simulink model "Drone2_simulink_old"  (R2024b)
settings: Solver=ode1be  StartTime=0.0  StopTime=1200  FixedStep=0.001  MaxStep=0.001  MinStep=0.00095  RelTol=1e-3
undefined symbols (not defined in the file): DiscIntNeverNeededParam, Environment, Newton, Raphson, Sim3dSensor, Vehicle, X, Y, Z
libraries: sm_lib x2953, nesl_utility x76, slpidlib x25, simulink x4, eeGeneralControl x4, matrix_library x3, rllib x2, sim3dlib x2, uavsim3dlib x2, dspstat3 x1, SignalEditorBlockLib x1, sharedutil x1
(part 1 of 21)
settings Model: Creator=Robotics  LastModifiedBy=admin
settings SolverCC: InitialStep=0.00095  MaxConsecutiveMinStep=5  ZeroCrossAlgorithm=Adaptive  EnableFixedStepZeroCrossing=on
settings OptimizationCC: ZeroExternalMemoryAtStartup=off  ZeroInternalMemoryAtStartup=off  InitFltsAndDblsToZero=on
settings DebuggingCC: AlgebraicLoopMsg=none
settings HardwareCC: ProdLongLongMode=on  TargetLongLongMode=on
settings RTWCC: TargetLang=C++  GenerateGPUCode=CUDA
settings GRTTargetCC: TargetLangStandard=C++11 (ISO)  CodeInterfacePackaging=C++ class
settings ExplorerConfigSet: InternalSimMechanicsExplorerSettings="<ExplorerConfiguration><canonicalview>default</canonicalview><AnimationSetting><BasePlaybackSpeed>1.0</BasePlaybackSpeed><PlaybackSpeedFactor>4.0</PlaybackSpeedFactor></AnimationSetting><TilePanel><TileInfo><Tiles Columns=\"2\" Count=\"4\" Rows=\"2\"><Column Weight=\"0.5\"/><Column Weight=\"0.5\"/><Row Weight=\"0.499\"/><Row Weight=\"0.501\"/><Tile Height=\"1\" Width=\"1\" X=\"0\" Y=\"0\"/><Tile Height=\"1\" Width=\"1\" X=\"0\" Y=\"1\"/><Tile Height=\"1\" Width=\"1\" X=\"1\" Y=\"0\"/><Tile Height=\"1\" Width=\"1\" X=\"1\" Y=\"1\"/></Tiles></TileInfo><SceneInfo><SceneViewer><BGColor><R>0.60000002384185791</R><G>0.60000002384185791</G><B>0.60000002384185791</B></BGColor><Camera><DoPerspective>off</DoPerspective><Position><X>-0.0113675484149264941</X><Y>-739.397084901340122</Y><Z>-0.0886193408787913639</Z></Position><Center><X>-0.0113675484149264941</X><Y>-5.95973369854618626e-06</Y><Z>-0.0886193408787913639</Z></Center><Up><X>0</X><Y>-0</Y><Z>1</Z></Up><ViewLimDist>1</ViewLimDist><YLim>0.330538852611916067</YLim><XLim>0.39239407649250857</XLim></Camera></SceneViewer><SceneViewer><BGColor><R>0.60000002384185791</R><G>0.60000002384185791</G><B>0.60000002384185791</B></BGColor><Camera><DoPerspective>off</DoPerspective><Position><X>-0.0123326458289036989</X><Y>0.0124784466883283152</Y><Z>779.159585012589673</Z></Position><Center><X>-0.0123326458289036989</X><Y>0.0124784466883283152</Y><Z>-5.16521799909241963e-06</Z></Center><Up><X>0</X><Y>1</Y><Z>-0</Z></Up><ViewLimDist>1</ViewLimDist><YLim>0.581385630746349302</YLim><XLim>0.686170250241330937</XLim></Camera></SceneViewer><SceneViewer><BGColor><R>0.60000002384185791</R><G>0.60000002384185791</G><B>0.60000002384185791</B></BGColor><Camera><DoPerspective>off</DoPerspective><Position><X>779.159585093457963</X><Y>0.0121540939985229218</Y><Z>-0.0872146397947211049</Z></Position><Center><X>-1.32520503939304035e-05</X><Y>0.0121540939985229218</Y><Z>-0.0872146397947211049</Z></Center><Up><X>-0</X><Y>0</Y><Z>1</Z></Up><ViewLimDist>1</ViewLimDist><YLim>0.279113201164486624</YLim><XLim>0.331344911323922742</XLim></Camera></SceneViewer><SceneViewer><BGColor><R>0.60000002384185791</R><G>0.60000002384185791</G><B>0.60000002384185791</B></BGColor><Camera><DoPerspective>off</DoPerspective><Position><X>436.235740070213467</X><Y>-436.218598621418209</Y><Z>436.235051594773893</Z></Position><Center><X>-13.3273814067072021</X><Y>13.344522855502376</Y><Z>-13.3280698821460408</Z></Center><Up><X>-0.408248290463863073</X><Y>0.408248290463863073</Y><Z>0.816496580927726145</Z></Up><ViewLimDist>1</ViewLimDist><YLim>0.509054047074245841</YLim><XLim>0.600802160209720437</XLim></Camera></SceneViewer></SceneInfo></TilePanel><MechEditorPanel><Cameras><Camera><Id>Camera1</Id><Value><Name>Camera1</Name><NativeCamera><PositionTrackingFeature>Physical_system.camera.F</PositionTrackingFeature><CenterTrackingFeature>Physical_system.camera.F</CenterTrackingFeature><UpVectorTrackingFeature>Physical_system.camera.F</UpVectorTrackingFeature><CenterTrackingOrigin>off</CenterTrackingOrigin><CenterTrackingDirection>+X</CenterTrackingDirection><UpVectorTrackingDirection>+Z</UpVectorTrackingDirection></NativeCamera></Value></Camera></Cameras><GfxPanelCameraMap/><VideoCreator><PlaybackSpeedRatio>8.0</PlaybackSpeedRatio><FrameRate>60</FrameRate><VideoFormat>Motion JPEG AVI</VideoFormat><FrameSize>[1920 1080]</FrameSize></VideoCreator></MechEditorPanel></ExplorerConfiguration>"

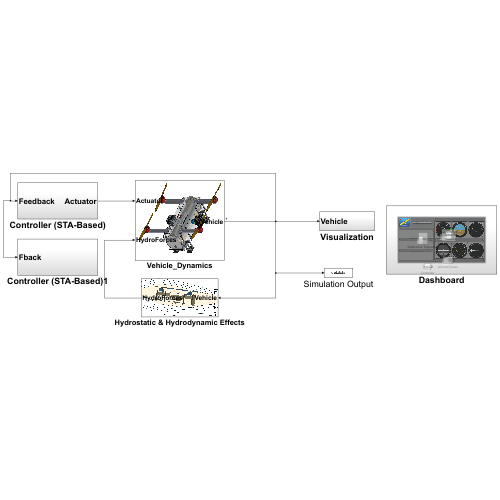
[thumbnail: Simulink's stored preview of the top-level diagram]
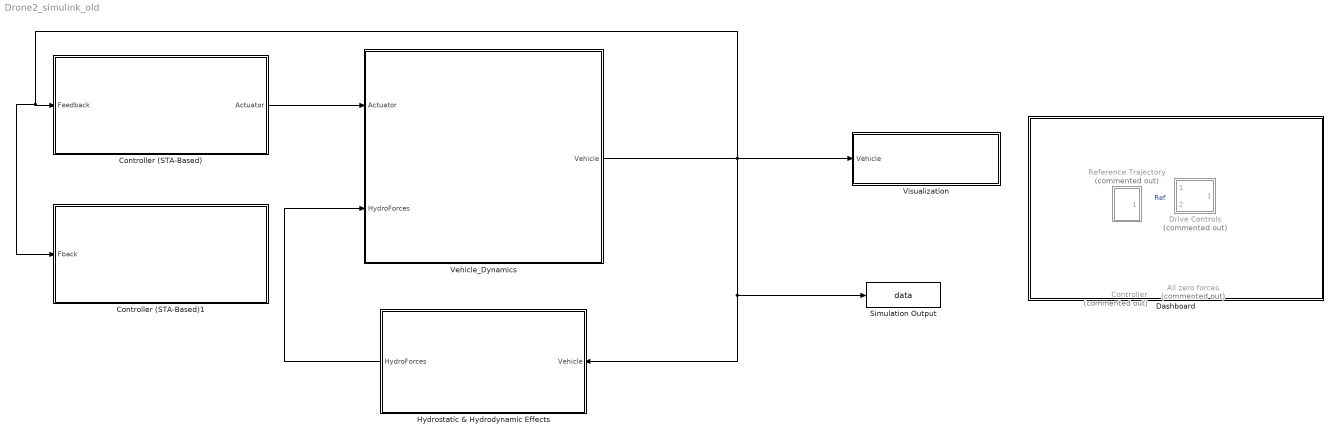
== system Drone2_simulink_old ==
  All zero forces : Subsystem  Commented=on
  Controller : Subsystem  Commented=on
  Controller (STA-Based) : Subsystem
  Controller (STA-Based)1 : Subsystem
  Dashboard : Subsystem
  Drive Controls : Subsystem  Commented=on
  Hydrostatic & Hydrodynamic Effects : Subsystem
      mask Display: image('Drage_new.png', [0,0,0,0,95,95])
  Reference Trajectory : Subsystem  Commented=on
  Simulation Output : ToWorkspace  VariableName=data  SaveFormat=Timeseries  SampleTime=-1
  Vehicle_Dynamics : Subsystem
      mask Display: image('Drone2_Assembly.PNG');
  Visualization : Subsystem
  wires:
  Reference Trajectory/1(Reference) -> Drive Controls/2(Reference)  "Ref"
  Vehicle_Dynamics/1(Vehicle) -> Hydrostatic & Hydrodynamic Effects/1(Vehicle), Simulation Output/1, Controller (STA-Based)1/1(Fback), Controller (STA-Based)/1(Feedback), Visualization/1(Vehicle)
  Hydrostatic & Hydrodynamic Effects/1(HydroForces) -> Vehicle_Dynamics/2(HydroForces)
  Controller (STA-Based)/1(Actuator) -> Vehicle_Dynamics/1(Actuator)

== system Drone2_simulink_old/All zero forces ==
  Constant : Constant  Value=0
  Constant3 : Constant  Value=0
  Constant9 : Constant  Value=0
  Out Bus Element : Outport  PortName=Actuator  Element=Aerial.MotorRB.Thrust
  Out Bus Element1 : Outport  PortName=Actuator  Element=Aerial.MotorRB.Torque
  Out Bus Element2 : Outport  PortName=Actuator  Element=Aerial.MotorRF.Torque
  Out Bus Element5 : Outport  PortName=Actuator  Element=Aerial.MotorRF.Thrust
  Out Bus Element3 : Outport  PortName=Actuator  Element=Aerial.MotorLF.Torque
  Out Bus Element6 : Outport  PortName=Actuator  Element=Aerial.MotorLF.Thrust
  Out Bus Element4 : Outport  PortName=Actuator  Element=Aerial.MotorLB.Torque
  Out Bus Element7 : Outport  PortName=Actuator  Element=Aerial.MotorLB.Thrust
  Out Bus Element8 : Outport  PortName=Actuator  Element=Underwater.ThrusterL.Thrust
  Out Bus Element9 : Outport  PortName=Actuator  Element=Underwater.ThrusterL.Torque
  Out Bus Element10 : Outport  PortName=Actuator  Element=Underwater.ThrusterR.Torque
  Out Bus Element11 : Outport  PortName=Actuator  Element=Underwater.ThrusterR.Thrust
  Out Bus Element12 : Outport  PortName=Actuator  Element=BuoyancyForce.SyringeFL.Force
  Out Bus Element13 : Outport  PortName=Actuator  Element=BuoyancyForce.SyringeFR.Force
  Out Bus Element14 : Outport  PortName=Actuator  Element=BuoyancyForce.SyringeB.Force
  wires:
  Constant/1 -> Out Bus Element9/1, Out Bus Element10/1
  Constant3/1 -> Out Bus Element11/1, Out Bus Element8/1
  Constant9/1 -> Out Bus Element13/1, Out Bus Element12/1, Out Bus Element14/1, Out Bus Element5/1, Out Bus Element2/1, Out Bus Element/1, Out Bus Element1/1, Out Bus Element6/1, Out Bus Element3/1, Out Bus Element7/1, Out Bus Element4/1

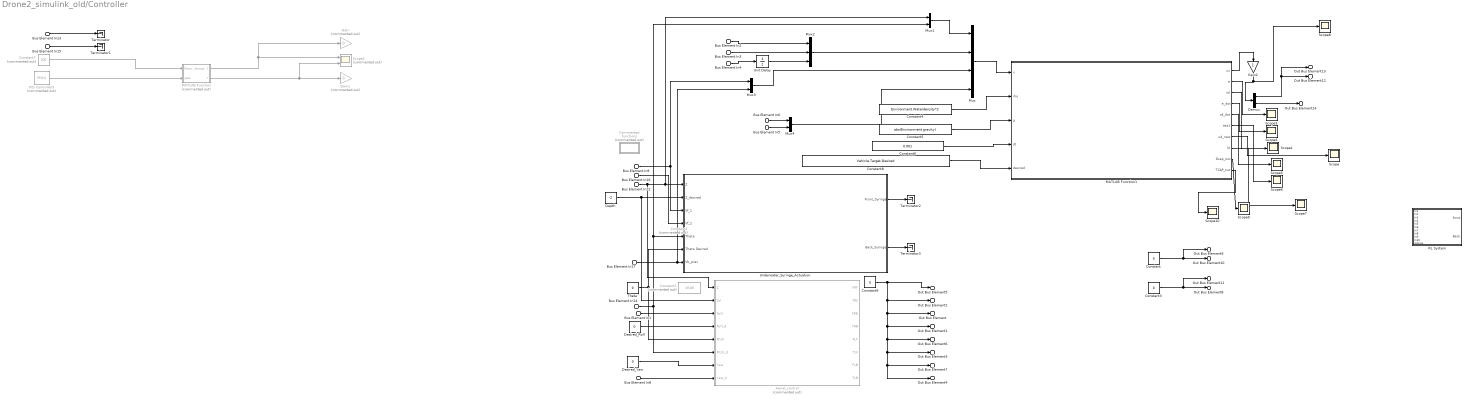
== system Drone2_simulink_old/Controller ==
  Bus Element In17 : Inport  PortName=Feedback  Element=Buoyancy.Syringe.SyringeB.Pose
  Bus Element In5 : Inport  PortName=Feedback  Element=Buoyancy.Syringe.SyringeB.Vel
  Bus Element In9 : Inport  PortName=Feedback  Element=Buoyancy.Syringe.SyringeFR.Pose
  Bus Element In6 : Inport  PortName=Feedback  Element=Buoyancy.Syringe.SyringeFR.Vel
  Bus Element In16 : Inport  PortName=Feedback  Element=Buoyancy.Syringe.SyringeFL.Pose
  Bus Element In14 : Inport  PortName=Feedback  Element=COM.Derived.Euler.theta
  Bus Element In8 : Inport  PortName=Feedback  Element=COM.Derived.Euler.psi
  Bus Element In1 : Inport  PortName=Feedback  Element=COM.Derived.Euler.phi
  Bus Element In13 : Inport  PortName=Feedback  Element=COM.World.Ve.Vz
  Bus Element In12 : Inport  PortName=Feedback  Element=COM.World.Xe.Z
  Bus Element In15 : Inport  PortName=Feedback  Element=COM.Body.wb.q
  Bus Element In2 : Inport  PortName=Feedback  Element=COM.Body.Vb.u
  Bus Element In3 : Inport  PortName=Feedback  Element=COM.Body.Vb.w
  Bus Element In4 : Inport  PortName=Feedback  Element=COM.Body.dwbdt.qdot
  Aerial_control : Subsystem  Commented=on
  Commented functions : Subsystem  Commented=on
  Constant : Constant  Value=0
  Constant1 : Constant  Commented=on  Value=19.85
  Constant2 : Constant  Commented=on  Value=20
  Constant3 : Constant  Value=0
  Constant4 : Constant  Value=Environment.Waterdensity*2
  Constant5 : Constant  Value=abs(Environment.gravity)
  Constant6 : Constant  Value=0.001
  Constant7 : Constant  Commented=on  Value=100
  Constant8 : Constant  Value=Vehicle.Target.Desired
  Constant9 : Constant  Value=0
  Demux : Demux  Outputs=2
  Depth : Constant  Value=-2
  Desired_Roll : Constant  Value=0
  Desired_Yaw : Constant  Value=0
  Gain : Gain  Commented=on  Gain=0
  Gain1 : Gain  Commented=on  Gain=0
  Gain2 : Gain
  MATLAB Function : MATLAB Function  Commented=on  TreatAsAtomicUnit=on
  MATLAB Function1 : MATLAB Function  TreatAsAtomicUnit=on
  Mux : Mux
  Mux1 : Mux  Inputs=2
  Mux2 : Mux  Inputs=3
  Mux3 : Mux  Inputs=2
  Mux4 : Mux  Inputs=2
  PID Controller3 : slpidlib/PID Controller  Commented=on  Controller=PD  Form=Parallel  TimeDomain=Discrete-time  UseExternalTs=off  SampleTime=0.001  IntegratorMethod=Forward Euler  FilterMethod=Backward Euler  ControllerParametersSource=internal  P=100  I=1  UseKiTs=off  D=5  UseExternalDerivativeSource=off  N=100  UseFilter=on  TunerSelectOption=Transfer Function Based (PID Tuner App)  InitialConditionSource=internal  InitialConditionForIntegrator=0  InitialConditionForFilter=0  DifferentiatorICPrevScaledInput=0  ExternalReset=none  TrackingMode=off  Kt=1  LimitOutput=off  SatLimitsSource=internal  UpperSaturationLimit=inf  LowerSaturationLimit=-inf  LinearizeAsGain=on  AntiWindupMode=none  Kb=1  LimitIntegrator=off  UpperIntegratorSaturationLimit=inf  LowerIntegratorSaturationLimit=-inf  POutMin=[]  POutMax=[]  IOutMin=[]  IOutMax=[]  DOutMin=[]  DOutMax=[]  NOutMin=[]  NOutMax=[]  SumOutMin=[]  SumOutMax=[]  SaturationOutMin=[]  SaturationOutMax=[]  PParamMin=[]  PParamMax=[]  IParamMin=[]  IParamMax=[]  DParamMin=[]  DParamMax=[]  NParamMin=[]  NParamMax=[]  KbParamMin=[]  KbParamMax=[]  KtParamMin=[]  KtParamMax=[]  KbOutMin=[]  KbOutMax=[]  KtOutMin=[]  KtOutMax=[]  IntegratorOutMin=[]  IntegratorOutMax=[]  FilterOutMin=[]  FilterOutMax=[]  SumI1OutMin=[]  SumI1OutMax=[]  SumI2OutMin=[]  SumI2OutMax=[]  SumI3OutMin=[]  SumI3OutMax=[]  SumI4OutMin=[]  SumI4OutMax=[]  SumDOutMin=[]  SumDOutMax=[]  DifferentiatorOutMin=[]  DifferentiatorOutMax=[]  FilterDiffOutCoefMin=[]  FilterDiffOutCoefMax=[]  ReciprocalOutMin=[]  ReciprocalOutMax=[]  SumDenOutMin=[]  SumDenOutMax=[]  SumNumOutMin=[]  SumNumOutMax=[]  DivideOutMin=[]  DivideOutMax=[]  UdiffTsProdOutMin=[]  UdiffTsProdOutMax=[]  NTsProdOutMin=[]  NTsProdOutMax=[]  UintegralTsProdOutMin=[]  UintegralTsProdOutMax=[]  UngainTsProdOutMin=[]  UngainTsProdOutMax=[]  ClampingZeroOutDataTypeStr=Inherit: Inherit via back propagation  ClampingZeroOutMin=[]  ClampingZeroOutMax=[]  FilterDenConstantOutDataTypeStr=Inherit: Inherit via back propagation  FilterDenConstantOutMin=[]  FilterDenConstantOutMax=[]  PCopyOutDataTypeStr=Inherit: Inherit via back propagation  PCopyOutMin=[]  PCopyOutMax=[]  NCopyOutDataTypeStr=Inherit: Inherit via back propagation  NCopyOutMin=[]  NCopyOutMax=[]  IntegratorContinuousStateAttributes=''  IntegratorStateMustResolveToSignalObject=off  IntegratorRTWStateStorageClass=Auto  FilterContinuousStateAttributes=''  FilterStateMustResolveToSignalObject=off  FilterRTWStateStorageClass=Auto  ParallelPVariant=InternalParameters  IdealPVariant=Disabled  IVariant=Disabled  DVariant=InternalParameters  IntegratorVariant=Disabled  SatVariant=Disabled  AWVariant=Disabled  PCopyVariant=Disabled  TRVariant=Disabled  FdbkBlocksVariant=Forward  IdealPFdbkVariant=Disabled  SatFdbkVariant=Disabled  DerivativeFilterVariant=BackwardEulerFilter  NVariant=InternalParameters  NCopyVariant=InternalParameters  FilterICVariant=InternalICsFilter  IntegratorICVariant=Disabled  ExternalResetVariant=Disabled  TRSumVariant=Passthrough  SumFdbkVariant=Disabled  SumVariant=Sum_PD  TsampFilterVariant=InternalTs  TsampNgainVariant=Passthrough  TsampIntegralVariant=Disabled_SignalSpec  ExternalSaturationOutDataTypeStr=Inherit: Same as second input  DerivativeSourceVariant=ErrorSignal
  RL System : Subsystem
  Scope{,1,3..10} (10 alike) : Scope
  Scope2 : Scope  Commented=on  NumInputPorts=2
  Terminator{,1..3} (4 alike) : Terminator
  Theta : Constant  Value=0
  Underwater_Syringe_Actuation : Subsystem
  Unit Delay : UnitDelay  SampleTime=-1  HasFrameUpgradeWarning=on
  Out Bus Element : Outport  PortName=Actuator  Element=Aerial.MotorRB.Thrust
  Out Bus Element1 : Outport  PortName=Actuator  Element=Aerial.MotorRB.Torque
  Out Bus Element2 : Outport  PortName=Actuator  Element=Aerial.MotorRF.Torque
  Out Bus Element5 : Outport  PortName=Actuator  Element=Aerial.MotorRF.Thrust
  Out Bus Element3 : Outport  PortName=Actuator  Element=Aerial.MotorLF.Torque
  Out Bus Element6 : Outport  PortName=Actuator  Element=Aerial.MotorLF.Thrust
  Out Bus Element4 : Outport  PortName=Actuator  Element=Aerial.MotorLB.Torque
  Out Bus Element7 : Outport  PortName=Actuator  Element=Aerial.MotorLB.Thrust
  Out Bus Element8 : Outport  PortName=Actuator  Element=Underwater.ThrusterL.Thrust
  Out Bus Element9 : Outport  PortName=Actuator  Element=Underwater.ThrusterL.Torque
  Out Bus Element10 : Outport  PortName=Actuator  Element=Underwater.ThrusterR.Torque
  Out Bus Element11 : Outport  PortName=Actuator  Element=Underwater.ThrusterR.Thrust
  Out Bus Element12 : Outport  PortName=Actuator  Element=BuoyancyForce.SyringeFL.Force
  Out Bus Element13 : Outport  PortName=Actuator  Element=BuoyancyForce.SyringeFR.Force
  Out Bus Element14 : Outport  PortName=Actuator  Element=BuoyancyForce.SyringeB.Force
  wires:
  Constant3/1 -> Out Bus Element8/1, Out Bus Element11/1
  Bus Element In15/1 -> Terminator1/1
  Bus Element In17/1 -> Mux3/2, Underwater_Syringe_Actuation/7(Vb_prev)
  Constant7/1 -> MATLAB Function/1(Forwardthrust)
  Constant/1 -> Out Bus Element10/1, Out Bus Element9/1
  PID Controller3/1 -> MATLAB Function/2(yaw)
  MATLAB Function/2(r) -> Gain1/1, Scope2/2
  Bus Element In16/1 -> Underwater_Syringe_Actuation/4(Vf_2)
  Bus Element In9/1 -> Mux3/1, Underwater_Syringe_Actuation/3(Vf_1)
  Bus Element In13/1 -> Terminator/1
  Bus Element In12/1 -> Mux1/1, Underwater_Syringe_Actuation/1(Z), Aerial_control/1(Z)
  Depth/1 -> Aerial_control/2(Zd), Underwater_Syringe_Actuation/2(Z_desired)
  Theta/1 -> Underwater_Syringe_Actuation/6(Theta Desired), Aerial_control/5(Pitch)
  Bus Element In14/1 -> Underwater_Syringe_Actuation/5(Theta), Mux1/2, Aerial_control/6(Pitch_d)
  Bus Element In1/1 -> Aerial_control/3(Roll)
  Desired_Roll/1 -> Aerial_control/4(Roll_d)
  Desired_Yaw/1 -> Aerial_control/7(Yaw)
  Bus Element In8/1 -> Aerial_control/8(Yaw_d)
  MATLAB Function/1(l) -> Scope2/1, Gain/1
  Constant9/1 -> Out Bus Element4/1, Out Bus Element7/1, Out Bus Element3/1, Out Bus Element6/1, Out Bus Element1/1, Out Bus Element/1, Out Bus Element2/1, Out Bus Element5/1
  Mux1/1 -> Mux/1
  Bus Element In2/1 -> Mux2/1
  Bus Element In3/1 -> Mux2/2
  Bus Element In4/1 -> Unit Delay/1
  Mux2/1 -> Mux/2
  Bus Element In5/1 -> Mux4/2
  Bus Element In6/1 -> Mux4/1
  Constant4/1 -> MATLAB Function1/2(rho)
  Constant5/1 -> MATLAB Function1/3(g)
  Constant6/1 -> MATLAB Function1/4(dt)
  Constant8/1 -> MATLAB Function1/5(desired)
  MATLAB Function1/1(uc) -> Gain2/1
  Mux/1 -> MATLAB Function1/1(x)
  Mux3/1 -> Mux/3
  Mux4/1 -> Mux/4
  Unit Delay/1 -> Mux2/3
  Underwater_Syringe_Actuation/2(Back_Syringe) -> Terminator3/1
  Underwater_Syringe_Actuation/1(Front_Syringe) -> Terminator2/1
  MATLAB Function1/3(vd) -> Scope1/1
  MATLAB Function1/2(e) -> Scope3/1
  MATLAB Function1/4(e_dot) -> Scope4/1
  MATLAB Function1/5(vd_dot) -> Scope5/1
  MATLAB Function1/6(eta1) -> Scope6/1
  Gain2/1 -> Scope8/1, Demux/1
  Demux/1 -> Out Bus Element13/1, Out Bus Element12/1
  Demux/2 -> Out Bus Element14/1
  MATLAB Function1/8(ld) -> Scope7/1
  MATLAB Function1/7(ud_new) -> Scope/1
  MATLAB Function1/9(Dcap_out) -> Scope9/1
  MATLAB Function1/10(TCAP_out) -> Scope10/1

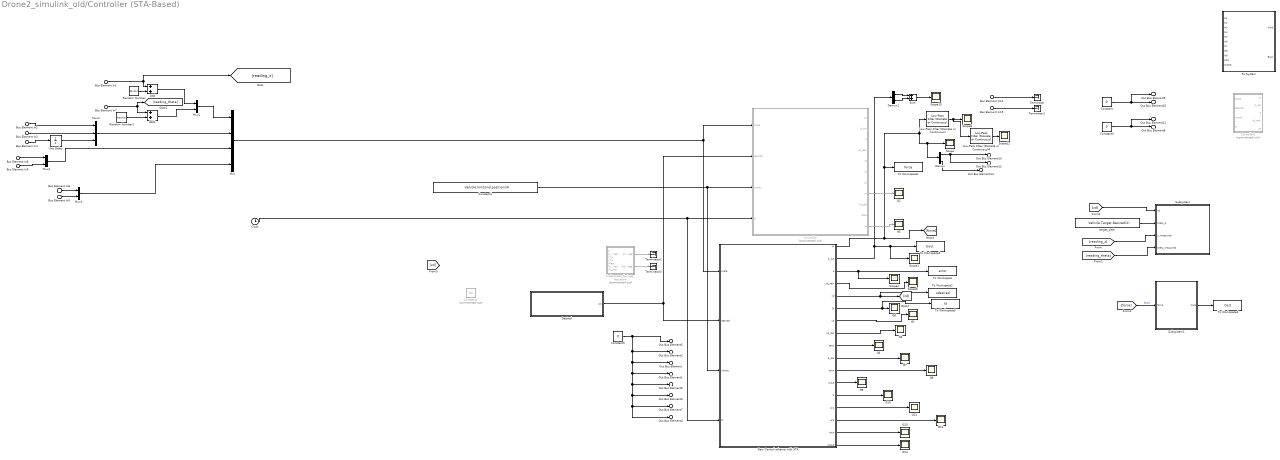
== system Drone2_simulink_old/Controller (STA-Based) ==
  Bus Element In5 : Inport  PortName=Feedback  Element=Buoyancy.Syringe.SyringeB.Vel
  Bus Element In9 : Inport  PortName=Feedback  Element=Buoyancy.Syringe.SyringeB.Pose
  Bus Element In6 : Inport  PortName=Feedback  Element=Buoyancy.Syringe.SyringeFR.Vel
  Bus Element In8 : Inport  PortName=Feedback  Element=Buoyancy.Syringe.SyringeFR.Pose
  Bus Element In13 : Inport  PortName=Feedback  Element=COM.World.Ve.Vz
  Bus Element In3 : Inport  PortName=Feedback  Element=COM.World.Ve.Vz
  Bus Element In1 : Inport  PortName=Feedback  Element=COM.World.Xe.Z
  Bus Element In15 : Inport  PortName=Feedback  Element=COM.Body.wb.q
  Bus Element In2 : Inport  PortName=Feedback  Element=COM.Body.Vb.u
  Bus Element In4 : Inport  PortName=Feedback  Element=COM.Body.dwbdt.qdot
  Bus Element In7 : Inport  PortName=Feedback  Element=COM.Derived.Euler.theta
  Add : Sum
  Add1 : Sum
  Clock : Clock
  Constant : Constant  Value=0
  Constant1 : Constant  Value=Vehicle.InitCond.position(3)
  Constant2 : Constant  Commented=on  Value=20
  Constant3 : Constant  Value=0
  Constant9 : Constant  Value=0
  Controller : MATLAB Function  Commented=on  TreatAsAtomicUnit=on  mask{m=7.61, IB=diag([0.09331 0.1703 0.2266]), Rsyringe=0.02, l=0.45, RG=[-0.002;0;-0.005], rb=[0;0;0.008], rho=Environment.Waterdensity, g=Environment.gravity, MaxBuoyancyVol=Vehicle.MaxBuoyancyForce/(abs(Environment.gravity*Environment.Waterdensity)), ZS=[0.033;0.033;0.033], Sden=1, dt=0.001, Ctrlchoice=Backsteppeng with disturbance compensator, k1e1=5, k1e2=2.5, k2e1=1, k2e2=10, k2e3=1, lambda11=5, lambda21=1, lambda12=2.5, lambda22=1, alpha1=3, KS11=01, KS12=100, KS13=10, k3e1=600, k3e2=600, TT=Vehicle.Syringe.Damping/Vehicle.Syringe.Stiffness, g1=5, g2=5, g3=5, d1=5, d2=5, sigma=0.5, sigma1=0.05, lb=0.1*eye(2), KS21=0.25, KS31=0.5, KS22=0.75, KS32=1, KS23=0.25, KS33=0.5, MaxIter=10, lambdaLM0=1e-3, tol_r=1e-6, tol_beta=1e-6, maxb=0.1, minb=0.01, alpha=0.960}
      mask prompts: m "Mass (Kg)"; IB "Inertia Matrix"; Rsyringe "Syringe radius (m)"; l "Length of Vehicle"; RG "Distance of CG from CO"; rb "Distance of CB from CO"; rho "Density"; g "Gravity"; MaxBuoyancyVol "Volume"; ZS "Syringe Z details"; Sden "Syringe Density multiplier"; dt "Sample time"; Ctrlchoice "Controller type"; k1e1 "K11"; k1e2 "K12"; k2e1 "K21"; k2e2 "K22"; k2e3 "K23"; lambda11 "lambda1-11"; lambda21 "lambda2-11"; lambda12 "lambda1-22"; lambda22 "lambda2-22"; alpha1 "STA alpha"; KS11 "KS1-11"; KS12 "KS1-22"; KS13 "KS1-33"; k3e1 "K31"; k3e2 "K32"; TT "Time constasnt"; g1 "Gamma1"; g2 "Gamma2"; g3 "Gamma3"; d1 "Delta1"; d2 "delta2"; sigma1 "T adptive sigma"; lb "Lambda b"; KS21 "KS2-11"; KS31 "KS3-11"; KS22 "KS2-22"; KS32 "KS3-22"; KS23 "KS2-33"; KS33 "KS3-33"; MaxIter "Max iteration"; lambdaLM0 "Lambda LM0"; tol_r "Relative Tolerance"; tol_beta "Beta tolerance"; maxb "Max"; minb "Min"; alpha "Smoothing constant"
      mask init:
      | % k1e1= 1; k1e2 = 1;
      | parameter.Backcomp.K1e = diag([k1e1 k1e2]); %2x2
      | 
      | % k2e1 = 10; k2e2 = 100; k2e3 =100;
      | parameter.Backcomp.K2eta1 = diag([k2e2 k2e3]); %2x2
      | 
      | % k3e1 = 200; k3e2 = 200;
      | parameter.Backcomp.K3eta2 = diag([k3e1 k3e2]);
      | 
      | % d1 = 5; d2 =5;
      | parameter.Backcomp.Del = diag([d1 d2]); %2x2
      | 
      | % g1 = 5; g2 = 5; g3 = 0.5;
      | parameter.Backcomp.Gama = diag([g1 g2 g3]);
      | 
      | parameter.Backcomp.sigma = sigma;
      | 
      | 
      | parameter.BackSTA.lambda1 = diag([lambda11 lambda12]); %2x2
      | 
      | 
      | parameter.BackSTA.lambda2 = diag([lambda21 lambda22]); %2x2
      | 
      | 
      | parameter.BackSTA.KS1= diag([KS11 KS12 KS13]);%3x3
      | 
      | 
      | parameter.BackSTA.KS2 = diag([KS21 KS22 KS23]); %2x2
      | 
      | 
      | parameter.BackSTA.KS3 = diag([KS31 KS32 KS33]);%3x3
      | parameter.BackSTA.alpha = alpha1;
      | 
      | 
      | parameter.opts.MaxIter = MaxIter;
      | parameter.opts.lambdaLM0 = lambdaLM0;
      | parameter.opts.tol_r = tol_r;
      | parameter.opts.tol_beta = 1e-6;
      | parameter.opts.regPI = tol_beta;
      | parameter.opts.beta_min = minb;
      | parameter.opts.beta_max = maxb;
      | parameter.opts.alpha = alpha;
      | parameter.Backcomp.lb=lb;
      | 
      | physical.m =m;
      | physical.IB = IB;
      | physical.Rsyringe = Rsyringe;
      | physical.RG =RG;
      | physical.rb =rb;
      | physical.l = l;
      | physical.ZS = ZS;
      | physical.Sden = Sden;
      | physical.maxb = maxb;
      | physical.minb = minb;
      | Env.rho = rho;
      | Env.g = g;
      | physical.MaxBuoyancyVol = MaxBuoyancyVol;
      | 
      | physical.TimeConstant = eye(2)*TT;
  Controller1 : MATLAB Function  Commented=on  TreatAsAtomicUnit=on  mask{m=7.61, IB=diag([0.09331 0.1703 0.2266]), Rsyringe=0.02, l=0.45, RG=[-0.002;0;-0.005], rb=[0;0;0.008], rho=Environment.Waterdensity, g=Environment.gravity, MaxBuoyancyVol=Vehicle.MaxBuoyancyForce/(abs(Environment.gravity*Environment.Waterdensity)), ZS=[0.0273;0.0273;0.0273], Sden=1, dt=0.001, Ctrlchoice=Backsteppeng with disturbance compensator, k1e1=5, k1e2=2.5, k2e1=10, k2e2=100, k2e3=100, k3e1=400, k3e2=400, g1=5, g2=5, g3=5, d1=5, d2=5, sigma=0.5, sigma1=0.05, lb=0.1*eye(2), MaxIter=10, lambdaLM0=1e-3, tol_r=1e-6, tol_beta=1e-6, maxb=0.1, minb=0.01, alpha=0.960}
      mask prompts: m "Mass (Kg)"; IB "Inertia Matrix"; Rsyringe "Syringe radius (m)"; l "Length of Vehicle"; RG "Distance of CG from CO"; rb "Distance of CB from CO"; rho "Density"; g "Gravity"; MaxBuoyancyVol "Volume"; ZS "Syringe Z details"; Sden "Syringe Density multiplier"; dt "Sample time"; Ctrlchoice "Controller type"; k1e1 "K11"; k1e2 "K12"; k2e1 "K21"; k2e2 "K22"; k2e3 "K23"; k3e1 "K31"; k3e2 "K32"; g1 "Gamma1"; g2 "Gamma2"; g3 "Gamma3"; d1 "Delta1"; d2 "delta2"; sigma1 "T adptive sigma"; lb "Lambda b"; MaxIter "Max iteration"; lambdaLM0 "Lambda LM0"; tol_r "Relative Tolerance"; tol_beta "Beta tolerance"; maxb "Max"; minb "Min"; alpha "Smoothing constant"
      mask init:
      | % k1e1= 1; k1e2 = 1;
      | parameter.Backcomp.K1e = diag([k1e1 k1e2]); %2x2
      | 
      | % k2e1 = 10; k2e2 = 100; k2e3 =100;
      | parameter.Backcomp.K2eta1 = diag([k2e1 k2e2 k2e3]); %3x3
      | 
      | % k3e1 = 200; k3e2 = 200;
      | parameter.Backcomp.K3eta2 = diag([k3e1 k3e2]);
      | 
      | % d1 = 5; d2 =5;
      | parameter.Backcomp.Del = diag([d1 d2]); %2x2
      | 
      | % g1 = 5; g2 = 5; g3 = 0.5;
      | parameter.Backcomp.Gama = diag([g1 g2 g3]);
      | 
      | parameter.Backcomp.sigma = sigma;
      | 
      | 
      | 
      | parameter.opts.MaxIter = MaxIter;
      | parameter.opts.lambdaLM0 = lambdaLM0;
      | parameter.opts.tol_r = tol_r;
      | parameter.opts.tol_beta = 1e-6;
      | parameter.opts.regPI = tol_beta;
      | parameter.opts.beta_min = minb;
      | parameter.opts.beta_max = maxb;
      | parameter.opts.alpha = alpha;
      | parameter.Backcomp.lb=lb;
      | 
      | physical.m =m;
      | physical.IB = IB;
      | physical.Rsyringe = Rsyringe;
      | physical.RG =RG;
      | physical.rb =rb;
      | physical.l = l;
      | physical.ZS = ZS;
      | physical.Sden = Sden;
      | physical.maxb = maxb;
      | physical.minb = minb;
      | Env.rho = rho;
      | Env.g = g;
      | physical.MaxBuoyancyVol = MaxBuoyancyVol;
  Demux : Demux  Outputs=2
  Demux1 : Demux  Outputs=2
  Desired : Subsystem
  G{1..14} (14 alike) : Scope
  Low-Pass Filter (Discrete or Continuous) : eeGeneralControl/Low-Pass Filter (Discrete or Continuous)  K=1  T=10  B=inf  A=-inf  init_option=Inherited from block input  x0=0  Ts=-1
  Low-Pass Filter (Discrete or Continuous)4 : eeGeneralControl/Low-Pass Filter (Discrete or Continuous)  K=1  T=10  B=inf  A=-inf  init_option=Inherited from block input  x0=0  Ts=-1
  Mux : Mux
  Mux1 : Mux  Inputs=2
  Mux2 : Mux  Inputs=3
  Mux3 : Mux  Inputs=2
  Mux4 : Mux  Inputs=2
  New Control scheme with STA : MATLAB Function  TreatAsAtomicUnit=on  mask{m=7.61, IB=diag([0.09331 0.1703 0.2266]), Rsyringe=0.02, l=0.45, RG=[-0.002;0;-0.005], rb=[0;0;0.008], rho=Environment.Waterdensity, g=Environment.gravity, MaxBuoyancyVol=Vehicle.MaxBuoyancyForce/(abs(Environment.gravity*Environment.Waterdensity)), ZS=[0.033;0.033;0.033], Sden=1, dt=0.001, k1e1=1, k1e2=0.5, k2e2=0.5, k2e3=0.5, k22e1=0.45, k22e2=0.3, k2z1=0.001, k2z2=0.005, k3e1=150, k3e2=150, k4e1=8, k4e2=10, k5e1=0.8, k5e2=1, TT=Vehicle.Syringe.Damping/Vehicle.Syringe.Stiffness, phi1f=0.05, phi1r=0.05, phid=0.01, phip=0.01, alpha0=0.75, alpha1=0.4286, lb=0.1*eye(2), K_Trim=0.002, K_Rate=0.05, EZDB=0, KP_Trim=0.0002, KP_Rate=0.05, ETDB=5, MaxIter=10, lambdaLM0=1e-3, tol_r=1e-6, tol_beta=1e-6, maxb=0.1, minb=0.01, alpha=0.960}
      mask prompts: m "Mass (Kg)"; IB "Inertia Matrix"; Rsyringe "Syringe radius (m)"; l "Length of Vehicle"; RG "Distance of CG from CO"; rb "Distance of CB from CO"; rho "Density"; g "Gravity"; MaxBuoyancyVol "Volume"; ZS "Syringe Z details"; Sden "Syringe Density multiplier"; dt "Sample time"; k1e1 "K11"; k1e2 "K12"; k2e2 "K22"; k2e3 "K23"; k22e1 "K221"; k22e2 "K222"; k3e1 "K1SF1"; k3e2 "K1SF2"; k4e1 "K2SF1"; k4e2 "K2SF2"; k5e1 "K3SF1"; k5e2 "K3SF2"; TT "Time constasnt"; phi1f "Front Syringe Saturation"; phi1r "Back Syringe Saturation"; phid "depth boundary layer"; phip "pitch boundary layer"; alpha0 "alpha"; lb "Lambda b"; EZDB "EZDB (in m)"; ETDB "ETDB (in degree)"; MaxIter "Max iteration"; lambdaLM0 "Lambda LM0"; tol_r "Relative Tolerance"; tol_beta "Beta tolerance"; maxb "Max"; minb "Min"; alpha "Smoothing constant"
      mask init:
      | % k1e1= 1; k1e2 = 1;
      | parameter.Backcomp.K1 = diag([k1e1 k1e2]); %2x2
      | 
      | % k2e1 = 10; k2e2 = 100; k2e3 =100;
      | parameter.Backcomp.K2 = diag([k2e2 k2e3]); %3x3
      | 
      | % k3e1 = 200; k3e2 = 200;
      | parameter.Backcomp.K22 = diag([k22e1 k22e2]);
      | parameter.Backcomp.K2Z = diag([k2z1 k2z2]);
      | 
      | % d1 = 5; d2 =5;
      | 
      | parameter.Backcomp.K1SF = diag([k3e1 k3e2]);
      | parameter.Backcomp.K2SF = diag([k4e1 k4e2]);
      | parameter.Backcomp.K3SF = diag([k5e1 k5e2]);
      | parameter.Backcomp.alpha = alpha0;
      | parameter.Backcomp.alpha1 = alpha1;
      | parameter.Backcomp.phisat = [phi1f; phi1r];
      | parameter.Backcomp.phisat1 = [phid;phip];
      | parameter.Backcomp.K_Trim = K_Trim;
      | parameter.Backcomp.K_Rate = K_Rate;
      | parameter.Backcomp.EZDB = EZDB;
      | parameter.Backcomp.KP_Trim = KP_Trim;
      | parameter.Backcomp.KP_Rate = KP_Rate;
      | parameter.Backcomp.ETDB = deg2rad(EZDB);
      | 
      | 
      | parameter.opts.MaxIter = MaxIter;
      | parameter.opts.lambdaLM0 = lambdaLM0;
      | parameter.opts.tol_r = tol_r;
      | parameter.opts.tol_beta = 1e-6;
      | parameter.opts.regPI = tol_beta;
      | parameter.opts.beta_min = minb;
      | parameter.opts.beta_max = maxb;
      | parameter.opts.alpha = alpha;
      | parameter.Backcomp.lb=lb;
      | 
      | physical.m =m;
      | physical.IB = IB;
      | physical.Rsyringe = Rsyringe;
      | physical.RG =RG;
      | physical.rb =rb;
      | physical.l = l;
      | physical.ZS = ZS;
      | physical.Sden = Sden;
      | physical.maxb = maxb;
      | physical.minb = minb;
      | Env.rho = rho;
      | Env.g = g;
      | physical.MaxBuoyancyVol = MaxBuoyancyVol;
      | 
      | physical.TimeConstant = eye(2)*TT;
  RL System : Subsystem
  Random Number : RandomNumber  Variance=(0.005)^2  Seed=42  SampleTime=0.1
  Random Number1 : RandomNumber  Variance=(0.0035)^2  Seed=42  SampleTime=0.1
  Scope{,1..2,5..6,12..13} (7 alike) : Scope
  Subsystem : Subsystem
  Subsystem1 : Subsystem
  Sum : Sum
  Terminator{,1..3} (4 alike) : Terminator
  To Workspace : ToWorkspace  VariableName=error  SaveFormat=Timeseries  SampleTime=-1
  To Workspace1 : ToWorkspace  VariableName=force  SaveFormat=Timeseries  SampleTime=-1
  To Workspace2 : ToWorkspace  VariableName=zdesired  SaveFormat=Timeseries  SampleTime=-1
  To Workspace3 : ToWorkspace  VariableName=bout  SaveFormat=Timeseries  SampleTime=-1
  To Workspace4 : ToWorkspace  VariableName=Cost  SaveFormat=Timeseries  SampleTime=-1
  To Workspace5 : ToWorkspace  VariableName=ld  SaveFormat=Timeseries  SampleTime=-1
  Underwater_Syringe_Actuation : Subsystem  Commented=on
  Unit Delay : UnitDelay  SampleTime=-1  HasFrameUpgradeWarning=on
  target_pitch : Constant  Value=Vehicle.Target.Desired(2)
  Out Bus Element : Outport  PortName=Actuator  Element=Aerial.MotorRB.Thrust
  Out Bus Element1 : Outport  PortName=Actuator  Element=Aerial.MotorRB.Torque
  Out Bus Element2 : Outport  PortName=Actuator  Element=Aerial.MotorRF.Torque
  Out Bus Element5 : Outport  PortName=Actuator  Element=Aerial.MotorRF.Thrust
  Out Bus Element3 : Outport  PortName=Actuator  Element=Aerial.MotorLF.Torque
  Out Bus Element6 : Outport  PortName=Actuator  Element=Aerial.MotorLF.Thrust
  Out Bus Element4 : Outport  PortName=Actuator  Element=Aerial.MotorLB.Torque
  Out Bus Element7 : Outport  PortName=Actuator  Element=Aerial.MotorLB.Thrust
  Out Bus Element8 : Outport  PortName=Actuator  Element=Underwater.ThrusterL.Thrust
  Out Bus Element9 : Outport  PortName=Actuator  Element=Underwater.ThrusterL.Torque
  Out Bus Element10 : Outport  PortName=Actuator  Element=Underwater.ThrusterR.Torque
  Out Bus Element11 : Outport  PortName=Actuator  Element=Underwater.ThrusterR.Thrust
  Out Bus Element12 : Outport  PortName=Actuator  Element=BuoyancyForce.SyringeFL.Force
  Out Bus Element14 : Outport  PortName=Actuator  Element=BuoyancyForce.SyringeB.Force
  Out Bus Element13 : Outport  PortName=Actuator  Element=BuoyancyForce.SyringeFR.Force
  wires:
  Underwater_Syringe_Actuation/1(Front_Syringe) -> Terminator2/1
  Underwater_Syringe_Actuation/2(Back_Syringe) -> Terminator3/1
  Unit Delay/1 -> Mux2/3
  Mux4/1 -> Mux/4
  Mux3/1 -> Mux/3
  Mux/1 -> Controller/1(state), New Control scheme with STA/1(state)
  Bus Element In6/1 -> Mux4/1
  Bus Element In5/1 -> Mux4/2
  Mux2/1 -> Mux/2
  Bus Element In4/1 -> Unit Delay/1
  Bus Element In3/1 -> Mux2/2
  Bus Element In2/1 -> Mux2/1
  Mux1/1 -> Mux/1
  Constant9/1 -> Out Bus Element5/1, Out Bus Element2/1, Out Bus Element/1, Out Bus Element1/1, Out Bus Element6/1, Out Bus Element3/1, Out Bus Element7/1, Out Bus Element4/1
  Bus Element In13/1 -> Terminator/1
  Constant/1 -> Out Bus Element9/1, Out Bus Element10/1
  Bus Element In15/1 -> Terminator1/1
  Constant3/1 -> Out Bus Element11/1, Out Bus Element8/1
  Add/1 -> Mux1/1
  Add1/1 -> Mux1/2
  Bus Element In8/1 -> Mux3/1
  Bus Element In9/1 -> Mux3/2
  New Control scheme with STA/1(uc) -> Demux/1, Scope/1, Low-Pass Filter (Discrete or Continuous)/1, To Workspace1/1, [force]
  Demux/1 -> Out Bus Element12/1, Out Bus Element13/1
  Demux/2 -> Out Bus Element14/1
  New Control scheme with STA/2(b_out) -> Demux1/1, Scope1/1, To Workspace3/1
  New Control scheme with STA/3(e) -> To Workspace/1, Scope2/1
  New Control scheme with STA/4(ud_new) -> Scope5/1
  Low-Pass Filter (Discrete or Continuous)/1 -> Low-Pass Filter (Discrete or Continuous)4/1, Scope6/1
  Low-Pass Filter (Discrete or Continuous)4/1 -> Scope12/1
  Demux1/1 -> Sum/1
  Demux1/2 -> Sum/2
  Sum/1 -> Scope13/1
  New Control scheme with STA/5(zd) -> To Workspace2/1, [zd]
  [reading_z] -> Subsystem/3(z_measured)
  [reading_theta] -> Subsystem/4(theta_measured)
  target_pitch/1 -> Subsystem/2(theta_d)
  [zd] -> Subsystem/1(zd)
  Constant1/1 -> New Control scheme with STA/3(initialz), Controller/3(initialz)
  Clock/1 -> New Control scheme with STA/4(tt), Controller/4(tt)
  New Control scheme with STA/7(vd) -> G1/1
  Controller/8(ur) -> G2/1
  New Control scheme with STA/8(vd_dot) -> G3/1
  New Control scheme with STA/9(eta1) -> G4/1
  Controller/11(je) -> G5/1
  New Control scheme with STA/6(ld) -> To Workspace5/1, G6/1
  New Control scheme with STA/10(e_dot) -> G7/1
  New Control scheme with STA/11(term) -> G8/1
  New Control scheme with STA/12(vzout) -> G9/1
  New Control scheme with STA/13(S) -> G10/1
  New Control scheme with STA/14(uc1) -> G11/1
  New Control scheme with STA/15(uc2) -> G12/1
  New Control scheme with STA/16(Aout) -> G13/1
  New Control scheme with STA/17(AAout) -> G14/1
  [force] -> Subsystem1/1(force)  "force"
  Subsystem1/1(Cost) -> To Workspace4/1
  Random Number/1 -> Add/2
  Bus Element In1/1 -> Add/1, [reading_z]
  Bus Element In7/1 -> [reading_theta], Add1/1
  Random Number1/1 -> Add1/2
  Desired/1(Zd) -> Controller/2(desired), New Control scheme with STA/2(desired)

== system Drone2_simulink_old/Controller (STA-Based)1 ==
  Bus Element In1 : Inport  PortName=Fback  Element=COM.Body.Vb.u

== system Drone2_simulink_old/Dashboard ==
  note: AUV DASHBOARD
  note: DEPTH (m)x100
  note: DEPTH (cm)
  note: DEPTH (cm)
  note: SPEED
  note: HEADING
  note: HORIZON
  note: MAIN PROPELLERS (N)
  note: VERTICAL THRUSTERS (N)
  note: HORIZONTAL THRUSTERS (N)
  note: VERTICAL SPEED (ft/min)x10
  note: TURN COORDINATOR
  note: DEPTH (ft)x100
  Airspeed Indicator : AirspeedIndicatorBlock  LabelPosition=Hide  ScaleMin=0  ScaleMax=9
  Altimeter : AltimeterBlock  LabelPosition=Hide
  Artificial Horizon : ArtificialHorizonBlock  LabelPosition=Hide
  Climb Rate Indicator : ClimbIndicatorBlock  LabelPosition=Hide
  Heading Indicator : HeadingIndicatorBlock  LabelPosition=Hide
  Turn Coordinator : TurnCoordinatorBlock  LabelPosition=Hide

== system Drone2_simulink_old/Drive Controls ==
  Bus Element In6 : Inport  PortName=VehicleFDBK
  Bus Element In1 : Inport  Port=2  PortName=Reference
  Thrust Controls : Subsystem
  Torque Controls : Subsystem
  Out Bus Element2 : Outport  PortName=ActuatorCMD  Element=Propellers.PPf
  Out Bus Element1 : Outport  PortName=ActuatorCMD  Element=Propellers.PPt
  Out Bus Element4 : Outport  PortName=ActuatorCMD  Element=Propellers.SPf
  Out Bus Element3 : Outport  PortName=ActuatorCMD  Element=Propellers.SPt
  Out Bus Element6 : Outport  PortName=ActuatorCMD  Element=Thrusters.BHTf
  Out Bus Element7 : Outport  PortName=ActuatorCMD  Element=Thrusters.BHTt
  Out Bus Element5 : Outport  PortName=ActuatorCMD  Element=Thrusters.BVTf
  Out Bus Element : Outport  PortName=ActuatorCMD  Element=Thrusters.BVTt
  Out Bus Element8 : Outport  PortName=ActuatorCMD  Element=Thrusters.SHTf
  Out Bus Element9 : Outport  PortName=ActuatorCMD  Element=Thrusters.SHTt
  Out Bus Element10 : Outport  PortName=ActuatorCMD  Element=Thrusters.SVTf
  Out Bus Element11 : Outport  PortName=ActuatorCMD  Element=Thrusters.SVTt
  wires:
  Torque Controls/1(BHTt) -> Out Bus Element7/1
  Torque Controls/2(BVTt) -> Out Bus Element/1
  Torque Controls/3(PPt) -> Out Bus Element1/1
  Torque Controls/4(SPt) -> Out Bus Element3/1
  Torque Controls/5(SHTt) -> Out Bus Element9/1
  Torque Controls/6(SVTt) -> Out Bus Element11/1
  Thrust Controls/3(BVTf) -> Out Bus Element5/1
  Thrust Controls/4(SVTf) -> Out Bus Element10/1
  Thrust Controls/5(BHTf) -> Out Bus Element6/1
  Thrust Controls/6(SHTf) -> Out Bus Element8/1
  Thrust Controls/1(PPf) -> Out Bus Element2/1
  Thrust Controls/2(SPf) -> Out Bus Element4/1
  Bus Element In6/1 -> Thrust Controls/2(VehicleFDBK)
  Bus Element In1/1 -> Thrust Controls/1(Reference)

== system Drone2_simulink_old/Hydrostatic & Hydrodynamic Effects ==
  Bus Element In6 : Inport  PortName=Vehicle  Element=COM.Body.Vb
  Bus Element In1 : Inport  PortName=Vehicle  Element=COM.Body.wb
  Bus Element In2 : Inport  PortName=Vehicle  Element=COM.Body.dwbdt
  Bus Element In7 : Inport  PortName=Vehicle  Element=COM.World.Xe.Z
  Bus Element In4 : Inport  PortName=Vehicle  Element=COM.World.R
  Bus Element In3 : Inport  PortName=Vehicle  Element=COM.Derived.Body.Abb
  Bus Element In5 : Inport  PortName=Vehicle  Element=COM.Derived.World.DCMbe
  Bus Element In10 : Inport  PortName=Vehicle  Element=Buoyancy.Syringe.SyringeB.Pose
  Bus Element In8 : Inport  PortName=Vehicle  Element=Buoyancy.Syringe.SyringeFR.Pose
  Bus Element In9 : Inport  PortName=Vehicle  Element=Buoyancy.Syringe.SyringeFL.Pose
  Added Mass Forces : Subsystem
  Buoyancy Force : Subsystem
  Drag Sub system : Subsystem
  Ocean Current : Subsystem
  Scope : Scope
  Scope1 : Scope  NumInputPorts=3
  Wind force : Subsystem
  syringe force block : MATLAB Function  TreatAsAtomicUnit=on  mask{FLy=0.027, FLz=0.033, FRy=-0.027, FRz=0.033, Ry=0, Rz=0.033, rho=Environment.Waterdensity, AS=pi()*Vehicle.Syringe.Radius^2, g=abs(Environment.gravity), l=0.45}
      mask prompts: rho "density"; AS "Area of Syringe"; g "gravity"; l "Length of drone"
  Bus Element Out3 : Outport  PortName=HydroForces  Element=Drag
  Bus Element Out4 : Outport  PortName=HydroForces  Element=BuoyancyForce
  Bus Element Out1 : Outport  PortName=HydroForces  Element=AddedMass
  Bus Element Out2 : Outport  PortName=HydroForces  Element=OceanCurrentForce
  Bus Element Out5 : Outport  PortName=HydroForces  Element=WindForce
  Bus Element Out6 : Outport  PortName=HydroForces  Element=syringe.FL
  Bus Element Out7 : Outport  PortName=HydroForces  Element=syringe.FR
  Bus Element Out8 : Outport  PortName=HydroForces  Element=syringe.R
  wires:
  Bus Element In2/1 -> Added Mass Forces/4(dwbdt)
  Bus Element In4/1 -> Wind force/3(Rotation Matrix), Ocean Current/3(Rotation Matrix)
  Bus Element In6/1 -> Ocean Current/1(Vb), Added Mass Forces/1(Vb), Wind force/1(Vb)
  Bus Element In3/1 -> Added Mass Forces/3(Abb)
  Bus Element In7/1 -> syringe force block/2(depth), Scope/1, Buoyancy Force/1(Z), Ocean Current/2(z), Wind force/2(z), Drag Sub system/1(Altitude)
  Bus Element In1/1 -> Added Mass Forces/2(wb), Drag Sub system/3(Omega_b)
  Drag Sub system/1(Drag) -> Bus Element Out3/1
  Wind force/1(Wind Force) -> Bus Element Out5/1
  Ocean Current/1(OceanCurrent) -> Bus Element Out2/1
  Added Mass Forces/1(AddedMass) -> Bus Element Out1/1
  Buoyancy Force/1(Buoyancy force) -> Bus Element Out4/1
  Bus Element In5/1 -> syringe force block/1(DCMbe)
  Bus Element In8/1 -> syringe force block/3(FLx)
  Bus Element In9/1 -> syringe force block/4(FRx)
  Bus Element In10/1 -> syringe force block/5(Rx)
  syringe force block/1(FL) -> Bus Element Out6/1, Scope1/1
  syringe force block/2(FR) -> Bus Element Out7/1, Scope1/2
  syringe force block/3(R) -> Scope1/3, Bus Element Out8/1
  Ocean Current/2(vr) -> [vr]
  [vr] -> Drag Sub system/2(vr)

== system Drone2_simulink_old/Reference Trajectory ==
  note: NOTE: Double-click on the Reference Trajectory block to choose the different Active Scenario available.
  Reference Trajectory : SignalEditorBlockLib/Signal Editor  FileName=RefTrajectory.mat  ActiveScenario=StraightDiveNTurn  ActiveSignal=Speed  IsBus=off  OutputBusObjectStr=Bus: BusObject  SampleTime=0  OutputAfterFinalValue=Holding final value  Unit=inherit  PreserveSignalName=on  ApplySigPropsToAllScenarios=on  ApplySigPropsToAllSignals=off
  deg2rad : Gain  Gain=pi/180
  Out Bus Element2 : Outport  PortName=Reference  Element=Speed
  Out Bus Element1 : Outport  PortName=Reference  Element=Depth
  Out Bus Element3 : Outport  PortName=Reference  Element=Heading
  wires:
  Reference Trajectory/1 -> Out Bus Element2/1
  Reference Trajectory/2 -> Out Bus Element1/1
  Reference Trajectory/3 -> deg2rad/1
  deg2rad/1 -> Out Bus Element3/1
